simulink model "TH3_6m"  (R2018b)
settings: Solver=VariableStepAuto  StartTime=0.0  StopTime=5  RelTol=1e-8
values from neighbouring files (symbols this model uses):
  G = [G1 G2 0 0]    [PCA_6.m]    (also in PCA_6b.m; PCA_6d.m = 1.0e+03 *[-6.4032   -2.2650   -1.0265   -0.2756]; TH3_7.m = [27 271 915]; TH3_7b.m = place(A, B, poles))
  G0 = Bnum*E    [PCA_6d.m]    (also in TH3_7b.m; TH3_8b.m)
settings Model: Creator=friedlan  LastModifiedBy=ohara
settings DebuggingCC: LibraryContextMissingDiagnostic=none
settings SFSimCC: SimUseLocalCustomCode=off
settings RTWCC: RTWUseLocalCustomCode=off

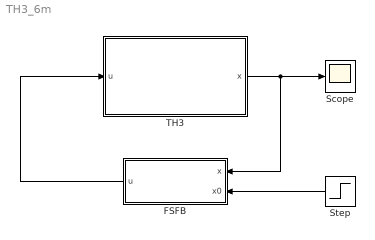
== system TH3_6m ==
  FSFB : Subsystem
  Scope : Scope
  Step : Step  SampleTime=0
  TH3 : Subsystem
  wires:
  TH3/1(x) -> FSFB/1(x), Scope/1
  FSFB/1(u) -> TH3/1(u)
  Step/1 -> FSFB/2(x0)

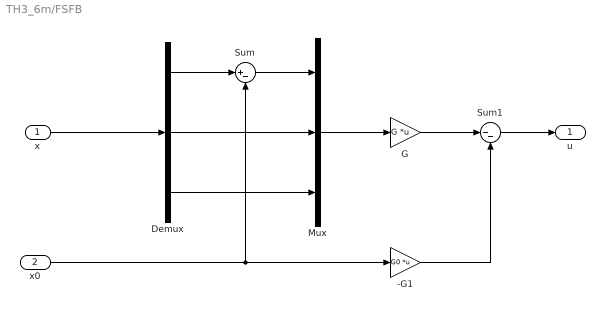
== system TH3_6m/FSFB ==
  x : Inport
  x0 : Inport  Port=2
  -G1 : Gain  Gain=G0  Multiplication=Matrix(K*u)
  Demux : Demux  Outputs=3
  G : Gain  Gain=G  Multiplication=Matrix(K*u)
  Mux : Mux  Inputs=3
  Sum : Sum  Inputs=|+-
  Sum1 : Sum  Inputs=|--
  u : Outport
  wires:
  x/1 -> Demux/1
  Mux/1 -> G/1
  Demux/2 -> Mux/2
  Demux/3 -> Mux/3
  Demux/1 -> Sum/1
  x0/1 -> -G1/1, Sum/2
  Sum/1 -> Mux/1
  G/1 -> Sum1/1
  -G1/1 -> Sum1/2
  Sum1/1 -> u/1

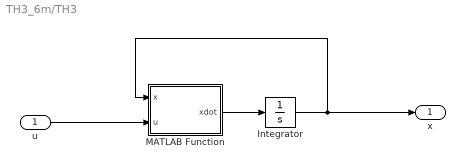
== system TH3_6m/TH3 ==
  u : Inport
  Integrator : Integrator  InitialCondition=[0;0;0]
  MATLAB Function : MATLAB Function  TreatAsAtomicUnit=on
  x : Outport
  wires:
  u/1 -> MATLAB Function/2(u)
  MATLAB Function/1(xdot) -> Integrator/1
  Integrator/1 -> x/1, MATLAB Function/1(x)

== matlab function TH3_6m/TH3/MATLAB Function ==
  data: x input; u input; xdot output
function xdot = TH3(x,u)
xdot1 = -3*x(1)+ x(2) ;
xdot2 = x(1)-2*x(2)+x(3);
xdot3 = x(2)-3*x(3) + u;
xdot = [xdot1; xdot2; xdot3];
